simulink model "sample_time_test"  (R2020b)
settings: Solver=VariableStepAuto  StartTime=0.0  StopTime=7  RelTol=1e-3
settings Model: Creator=abdullah  LastModifiedBy=abdullah

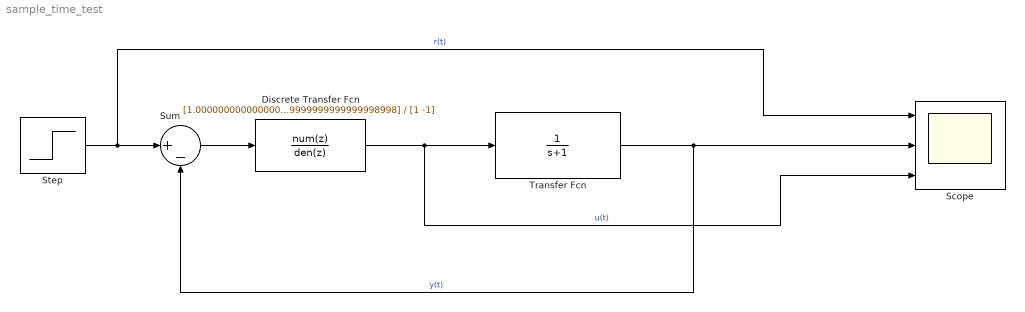
== system sample_time_test ==
  Discrete Transfer Fcn : DiscreteTransferFcn  Numerator=[1.00000000000000000001 -0.999999999999999999998998]  Denominator=[1 -1]  SampleTime=1e-6
  Scope : Scope  NumInputPorts=3
  Step : Step  SampleTime=0
  Sum : Sum  Inputs=|+-
  Transfer Fcn : TransferFcn  Denominator=[1 1]
  wires:
  Discrete Transfer Fcn/1 -> Scope/3, Transfer Fcn/1  "u(t)"
  Transfer Fcn/1 -> Sum/2, Scope/2  "y(t)"
  Step/1 -> Scope/1, Sum/1  "r(t)"
  Sum/1 -> Discrete Transfer Fcn/1
